simulink model "lsbexp"  (R2021b)
settings: Solver=FixedStepAuto  StartTime=0.0  StopTime=8  FixedStep=1/100  RelTol=1e-3
settings Model: Creator=sucho  LastModifiedBy=sucho
settings DebuggingCC: UnconnectedInputMsg=none  UnconnectedOutputMsg=none  UnconnectedLineMsg=none
settings ModelReferenceCC: EnableRefExpFcnMdlSchedulingChecks=off
settings RTWCC: DLArmComputeVersion=20.02.1

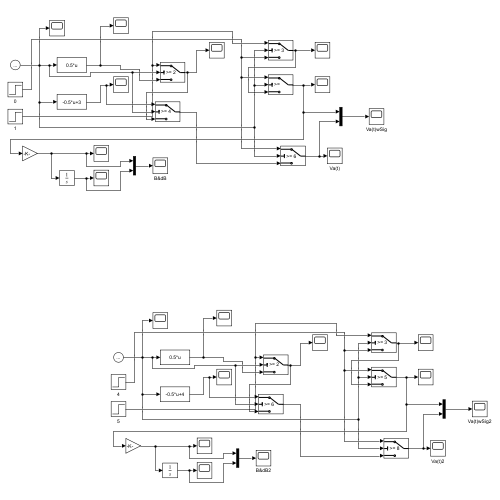
[thumbnail: Simulink's stored preview of the top-level diagram]
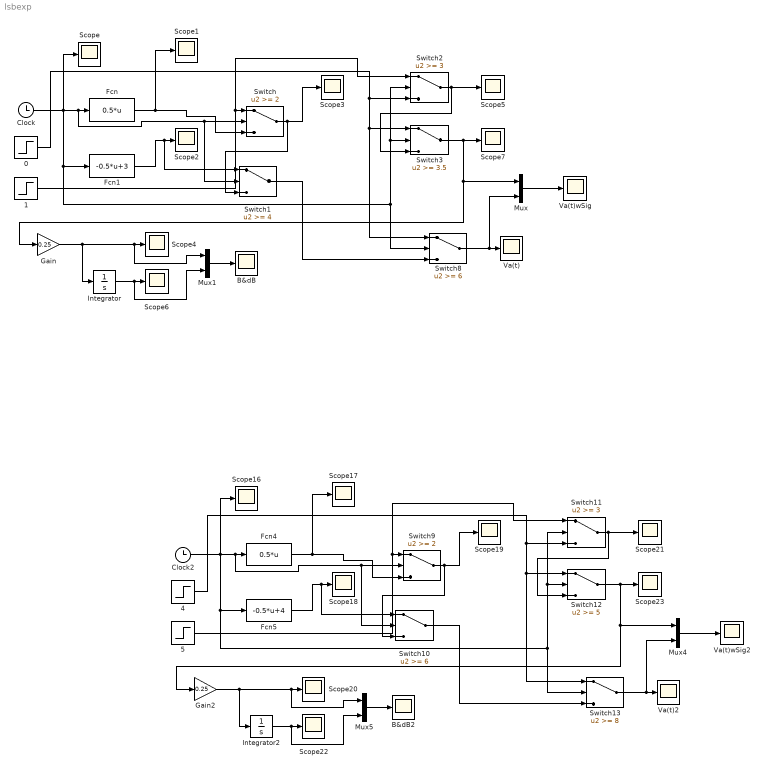
== system lsbexp ==
  0 : Step  Time=0  After=0  SampleTime=0
  1 : Step  Time=0  SampleTime=0
  4 : Step  Time=0  After=0  SampleTime=0
  5 : Step  Time=0  SampleTime=0
  B&dB : Scope
  B&dB2 : Scope
  Clock : Clock
  Clock2 : Clock
  Fcn : Fcn  Expr=0.5*u
  Fcn1 : Fcn  Expr=-0.5*u+3
  Fcn4 : Fcn  Expr=0.5*u
  Fcn5 : Fcn  Expr=-0.5*u+4
  Gain : Gain  Gain=0.25
  Gain2 : Gain  Gain=0.25
  Integrator : Integrator
  Integrator2 : Integrator
  Mux{,1,4..5} (4 alike) : Mux  Inputs=2
  Scope{,1..7,16..23} (16 alike) : Scope
  Switch : Switch  Threshold=2
  Switch1 : Switch  Threshold=4
  Switch10 : Switch  Threshold=6
  Switch11 : Switch  Threshold=3
  Switch12 : Switch  Threshold=5
  Switch13 : Switch  Threshold=8
  Switch2 : Switch  Threshold=3
  Switch3 : Switch  Threshold=3.5
  Switch8 : Switch  Threshold=6
  Switch9 : Switch  Threshold=2
  Va(t) : Scope
  Va(t)2 : Scope
  Va(t)wSig : Scope
  Va(t)wSig2 : Scope
  wires:
  Fcn/1 -> Switch/3, Scope1/1
  Clock/1 -> Scope/1, Fcn1/1, Switch8/2, Switch3/2, Switch2/2, Switch1/2, Switch/2, Fcn/1
  Fcn1/1 -> Switch1/1, Scope2/1
  1/1 -> Switch2/1, Switch/1
  Switch/1 -> Switch1/3, Scope3/1
  Switch1/1 -> Switch8/3
  0/1 -> Switch3/1, Switch8/1, Switch2/3
  Switch2/1 -> Switch3/3, Scope5/1
  Switch3/1 -> Gain/1, Mux/1, Scope7/1
  Mux/1 -> Va(t)wSig/1
  Gain/1 -> Integrator/1, Mux1/1, Scope4/1
  Integrator/1 -> Mux1/2, Scope6/1
  Mux1/1 -> B&dB/1
  Switch8/1 -> Mux/2, Va(t)/1
  Switch11/1 -> Switch12/3, Scope21/1
  Switch9/1 -> Switch10/3, Scope19/1
  Switch10/1 -> Switch13/3
  4/1 -> Switch12/1, Switch13/1, Switch11/3
  5/1 -> Switch11/1, Switch9/1
  Clock2/1 -> Scope16/1, Fcn5/1, Switch13/2, Switch12/2, Switch11/2, Switch10/2, Switch9/2, Fcn4/1
  Gain2/1 -> Integrator2/1, Mux5/1, Scope20/1
  Mux5/1 -> B&dB2/1
  Mux4/1 -> Va(t)wSig2/1
  Switch12/1 -> Gain2/1, Mux4/1, Scope23/1
  Fcn4/1 -> Switch9/3, Scope17/1
  Switch13/1 -> Mux4/2, Va(t)2/1
  Integrator2/1 -> Mux5/2, Scope22/1
  Fcn5/1 -> Switch10/1, Scope18/1
